simulink model "PID"  (R2023b)
settings: Solver=VariableStepAuto  StartTime=0.0  StopTime=10.0  RelTol=1e-3
values from neighbouring files (symbols this model uses):
  b_a = J_nom*(2*zeta_PID+1)*w_n_PID    (= 0.03957)    [Controlador.m]    (also in varLC.m = 0.0916527777778)
  K_a = J_nom*(2*zeta_PID+1)*w_n_PID^2    (= 31.656)    [Controlador.m]    (also in varLC.m = 73.3222222222)
  K_ai = J_nom*w_n_PID^3    (= 10129.92)    [Controlador.m]    (also in varLC.m = 23463.1111111)
settings Model: Creator=gonza  LastModifiedBy=gonza

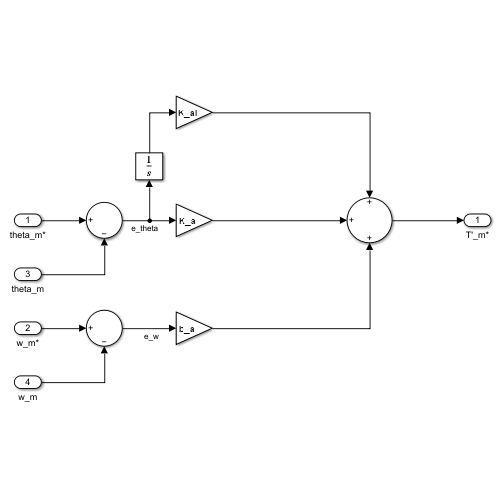
[thumbnail: Simulink's stored preview of the top-level diagram]
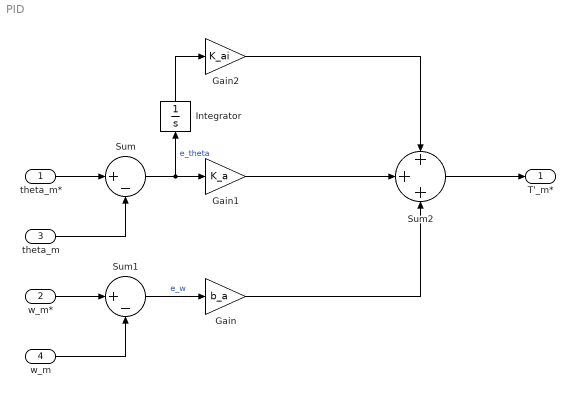
== system PID ==
  theta_m* : Inport
  w_m* : Inport  Port=2
  theta_m : Inport  Port=3
  w_m : Inport  Port=4
  Gain : Gain  Gain=b_a
  Gain1 : Gain  Gain=K_a
  Gain2 : Gain  Gain=K_ai
  Integrator : Integrator
  Sum : Sum  Inputs=|+-
  Sum1 : Sum  Inputs=|+-
  Sum2 : Sum  Inputs=+++
  T'_m* : Outport
  wires:
  w_m*/1 -> Sum1/1
  w_m/1 -> Sum1/2
  theta_m*/1 -> Sum/1
  theta_m/1 -> Sum/2
  Sum1/1 -> Gain/1  "e_w"
  Gain1/1 -> Sum2/2
  Gain2/1 -> Sum2/1
  Gain/1 -> Sum2/3
  Sum/1 -> Integrator/1, Gain1/1  "e_theta"
  Integrator/1 -> Gain2/1
  Sum2/1 -> T'_m*/1
